simulink model "T02_SimModel_01"  (R2016b)
settings: Solver=ode1  StartTime=0  StopTime=200  FixedStep=0.02  RelTol=1e-3
libraries: dspstat3 x2, simulink x1
settings Model: Creator=Maksim  LastModifiedBy=Maksim

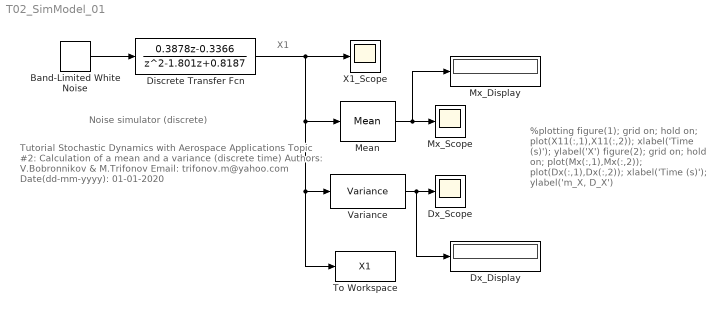
== system T02_SimModel_01 ==
  note: Tutorial Stochastic Dynamics with Aerospace Applications
      | Topic #2: Calculation of a mean and a variance (discrete time)
      | Authors: V.Bobronnikov & M.Trifonov
      | Email: trifonov.m@yahoo.com
      | Date(dd-mm-yyyy): 01-01-2020
  note: %plotting
      | figure(1); grid on; hold on;
      | plot(X11(:,1),X11(:,2));
      | xlabel('Time (s)'); ylabel('X')
      | figure(2); grid on; hold on;
      | plot(Mx(:,1),Mx(:,2));
      | plot(Dx(:,1),Dx(:,2));
      | xlabel('Time (s)'); ylabel('m_X, D_X')
  note: X1
  note: Noise simulator (discrete)
  Band-Limited White Noise : simulink/Sources/Band-Limited White Noise  Cov=[1]  Ts=0.2  seed=[23346]
  Discrete Transfer Fcn : DiscreteTransferFcn  Numerator=[0.3878 -0.3366]  Denominator=[1 -1.801 0.8187]
  Dx_Display : Display
  Dx_Scope : Scope
  Mean : dspstat3/Mean  run=on  reset_popup=None  InputProcessing=Inherited (this choice will be removed - see release notes)  directionMode=Each column  dimension=1  roiEnable=off  roiType=Rectangles  roiPortion=Entire ROI  roiOutput=Individual statistics for each ROI  roiFlag=off  outputDataTypeStr=Inherit: Same as accumulator  outputLastDataTypeStr=Inherit: Same as accumulator  outputMin=[]  outputMax=[]  roundingMode=Floor  overflowMode=off
  Mx_Display : Display
  Mx_Scope : Scope
  To Workspace : ToWorkspace  VariableName=X1  SampleTime=-1
  Variance : dspstat3/Variance  run=on  reset_popup=None  InputProcessing=Columns as channels (frame based)  directionMode=Each column  dimension=1  roiEnable=off  roiType=Rectangles  roiPortion=Entire ROI  roiOutput=Individual statistics for each ROI  roiFlag=off  roundingMode=Floor  overflowMode=off
  X1_Scope : Scope
  wires:
  Band-Limited White Noise/1 -> Discrete Transfer Fcn/1
  Discrete Transfer Fcn/1 -> X1_Scope/1, To Workspace/1, Variance/1, Mean/1
  Mean/1 -> Mx_Display/1, Mx_Scope/1
  Variance/1 -> Dx_Display/1, Dx_Scope/1
